simulink model "dmt_sim"  (Simulink 6.0)
settings: Solver=ode45  StartTime=0.0  StopTime=inf  RelTol=1e-3
model workspace: external: M-Code (data not in the file)
undefined symbols (not defined in the file or in its folder): b, slcm
libraries: commdigbbndam2 x512, simulink x35, dspxfrm3 x2, commchan2 x1, commrandsrc2 x1, dspsigattribs x1, dspsrcs4 x1, dspindex x1, commsink2 x1, dspsnks4 x1
(part 5 of 5)

== system dmt_sim/DMT Modulator/Modulator Bank 6 ==
  In1 : Inport  LatchInput=off
  Demux1 : Demux  Outputs=b(offset+1:offset+16)
  Matrix Concatenation : simulink/Math Operations/Matrix Concatenation  numInports=16  catMethod=Vertical
  Rectangular QAM Modulator Baseband1 : commdigbbndam2/Rectangular QAM Modulator Baseband  M=2^b(offset+1)  InType=Bit  Enc=Binary  PowType=Min. distance between symbols  MinDist=2  AvgPow=1  PeakPow=1  Ph=0  numSamp=1
  Rectangular QAM Modulator Baseband10 : commdigbbndam2/Rectangular QAM Modulator Baseband  M=2^b(offset+10)  InType=Bit  Enc=Binary  PowType=Min. distance between symbols  MinDist=2  AvgPow=1  PeakPow=1  Ph=0  numSamp=1
  Rectangular QAM Modulator Baseband11 : commdigbbndam2/Rectangular QAM Modulator Baseband  M=2^b(offset+11)  InType=Bit  Enc=Binary  PowType=Min. distance between symbols  MinDist=2  AvgPow=1  PeakPow=1  Ph=0  numSamp=1
  Rectangular QAM Modulator Baseband12 : commdigbbndam2/Rectangular QAM Modulator Baseband  M=2^b(offset+12)  InType=Bit  Enc=Binary  PowType=Min. distance between symbols  MinDist=2  AvgPow=1  PeakPow=1  Ph=0  numSamp=1
  Rectangular QAM Modulator Baseband13 : commdigbbndam2/Rectangular QAM Modulator Baseband  M=2^b(offset+13)  InType=Bit  Enc=Binary  PowType=Min. distance between symbols  MinDist=2  AvgPow=1  PeakPow=1  Ph=0  numSamp=1
  Rectangular QAM Modulator Baseband14 : commdigbbndam2/Rectangular QAM Modulator Baseband  M=2^b(offset+14)  InType=Bit  Enc=Binary  PowType=Min. distance between symbols  MinDist=2  AvgPow=1  PeakPow=1  Ph=0  numSamp=1
  Rectangular QAM Modulator Baseband15 : commdigbbndam2/Rectangular QAM Modulator Baseband  M=2^b(offset+15)  InType=Bit  Enc=Binary  PowType=Min. distance between symbols  MinDist=2  AvgPow=1  PeakPow=1  Ph=0  numSamp=1
  Rectangular QAM Modulator Baseband16 : commdigbbndam2/Rectangular QAM Modulator Baseband  M=2^b(offset+16)  InType=Bit  Enc=Binary  PowType=Min. distance between symbols  MinDist=2  AvgPow=1  PeakPow=1  Ph=0  numSamp=1
  Rectangular QAM Modulator Baseband2 : commdigbbndam2/Rectangular QAM Modulator Baseband  M=2^b(offset+2)  InType=Bit  Enc=Binary  PowType=Min. distance between symbols  MinDist=2  AvgPow=1  PeakPow=1  Ph=0  numSamp=1
  Rectangular QAM Modulator Baseband3 : commdigbbndam2/Rectangular QAM Modulator Baseband  M=2^b(offset+3)  InType=Bit  Enc=Binary  PowType=Min. distance between symbols  MinDist=2  AvgPow=1  PeakPow=1  Ph=0  numSamp=1
  Rectangular QAM Modulator Baseband4 : commdigbbndam2/Rectangular QAM Modulator Baseband  M=2^b(offset+4)  InType=Bit  Enc=Binary  PowType=Min. distance between symbols  MinDist=2  AvgPow=1  PeakPow=1  Ph=0  numSamp=1
  Rectangular QAM Modulator Baseband5 : commdigbbndam2/Rectangular QAM Modulator Baseband  M=2^b(offset+5)  InType=Bit  Enc=Binary  PowType=Min. distance between symbols  MinDist=2  AvgPow=1  PeakPow=1  Ph=0  numSamp=1
  Rectangular QAM Modulator Baseband6 : commdigbbndam2/Rectangular QAM Modulator Baseband  M=2^b(offset+6)  InType=Bit  Enc=Binary  PowType=Min. distance between symbols  MinDist=2  AvgPow=1  PeakPow=1  Ph=0  numSamp=1
  Rectangular QAM Modulator Baseband7 : commdigbbndam2/Rectangular QAM Modulator Baseband  M=2^b(offset+7)  InType=Bit  Enc=Binary  PowType=Min. distance between symbols  MinDist=2  AvgPow=1  PeakPow=1  Ph=0  numSamp=1
  Rectangular QAM Modulator Baseband8 : commdigbbndam2/Rectangular QAM Modulator Baseband  M=2^b(offset+8)  InType=Bit  Enc=Binary  PowType=Min. distance between symbols  MinDist=2  AvgPow=1  PeakPow=1  Ph=0  numSamp=1
  Rectangular QAM Modulator Baseband9 : commdigbbndam2/Rectangular QAM Modulator Baseband  M=2^b(offset+9)  InType=Bit  Enc=Binary  PowType=Min. distance between symbols  MinDist=2  AvgPow=1  PeakPow=1  Ph=0  numSamp=1
  Out1 : Outport
  wires:
  Rectangular QAM Modulator Baseband16/1 -> Matrix Concatenation/16
  Rectangular QAM Modulator Baseband15/1 -> Matrix Concatenation/15
  Rectangular QAM Modulator Baseband14/1 -> Matrix Concatenation/14
  Rectangular QAM Modulator Baseband13/1 -> Matrix Concatenation/13
  Rectangular QAM Modulator Baseband12/1 -> Matrix Concatenation/12
  Rectangular QAM Modulator Baseband11/1 -> Matrix Concatenation/11
  Rectangular QAM Modulator Baseband10/1 -> Matrix Concatenation/10
  Rectangular QAM Modulator Baseband9/1 -> Matrix Concatenation/9
  Rectangular QAM Modulator Baseband8/1 -> Matrix Concatenation/8
  Rectangular QAM Modulator Baseband7/1 -> Matrix Concatenation/7
  Rectangular QAM Modulator Baseband6/1 -> Matrix Concatenation/6
  Rectangular QAM Modulator Baseband5/1 -> Matrix Concatenation/5
  Rectangular QAM Modulator Baseband4/1 -> Matrix Concatenation/4
  Rectangular QAM Modulator Baseband3/1 -> Matrix Concatenation/3
  Rectangular QAM Modulator Baseband2/1 -> Matrix Concatenation/2
  Demux1/16 -> Rectangular QAM Modulator Baseband16/1
  Demux1/15 -> Rectangular QAM Modulator Baseband15/1
  Demux1/14 -> Rectangular QAM Modulator Baseband14/1
  Demux1/13 -> Rectangular QAM Modulator Baseband13/1
  Demux1/12 -> Rectangular QAM Modulator Baseband12/1
  Demux1/11 -> Rectangular QAM Modulator Baseband11/1
  Demux1/10 -> Rectangular QAM Modulator Baseband10/1
  Demux1/9 -> Rectangular QAM Modulator Baseband9/1
  Demux1/8 -> Rectangular QAM Modulator Baseband8/1
  Demux1/7 -> Rectangular QAM Modulator Baseband7/1
  Demux1/6 -> Rectangular QAM Modulator Baseband6/1
  Demux1/5 -> Rectangular QAM Modulator Baseband5/1
  Demux1/4 -> Rectangular QAM Modulator Baseband4/1
  Demux1/3 -> Rectangular QAM Modulator Baseband3/1
  Matrix Concatenation/1 -> Out1/1
  In1/1 -> Demux1/1
  Demux1/2 -> Rectangular QAM Modulator Baseband2/1
  Demux1/1 -> Rectangular QAM Modulator Baseband1/1
  Rectangular QAM Modulator Baseband1/1 -> Matrix Concatenation/1

== system dmt_sim/DMT Modulator/Modulator Bank 7 ==
  In1 : Inport  LatchInput=off
  Demux1 : Demux  Outputs=b(offset+1:offset+16)
  Matrix Concatenation : simulink/Math Operations/Matrix Concatenation  numInports=16  catMethod=Vertical
  Rectangular QAM Modulator Baseband1 : commdigbbndam2/Rectangular QAM Modulator Baseband  M=2^b(offset+1)  InType=Bit  Enc=Binary  PowType=Min. distance between symbols  MinDist=2  AvgPow=1  PeakPow=1  Ph=0  numSamp=1
  Rectangular QAM Modulator Baseband10 : commdigbbndam2/Rectangular QAM Modulator Baseband  M=2^b(offset+10)  InType=Bit  Enc=Binary  PowType=Min. distance between symbols  MinDist=2  AvgPow=1  PeakPow=1  Ph=0  numSamp=1
  Rectangular QAM Modulator Baseband11 : commdigbbndam2/Rectangular QAM Modulator Baseband  M=2^b(offset+11)  InType=Bit  Enc=Binary  PowType=Min. distance between symbols  MinDist=2  AvgPow=1  PeakPow=1  Ph=0  numSamp=1
  Rectangular QAM Modulator Baseband12 : commdigbbndam2/Rectangular QAM Modulator Baseband  M=2^b(offset+12)  InType=Bit  Enc=Binary  PowType=Min. distance between symbols  MinDist=2  AvgPow=1  PeakPow=1  Ph=0  numSamp=1
  Rectangular QAM Modulator Baseband13 : commdigbbndam2/Rectangular QAM Modulator Baseband  M=2^b(offset+13)  InType=Bit  Enc=Binary  PowType=Min. distance between symbols  MinDist=2  AvgPow=1  PeakPow=1  Ph=0  numSamp=1
  Rectangular QAM Modulator Baseband14 : commdigbbndam2/Rectangular QAM Modulator Baseband  M=2^b(offset+14)  InType=Bit  Enc=Binary  PowType=Min. distance between symbols  MinDist=2  AvgPow=1  PeakPow=1  Ph=0  numSamp=1
  Rectangular QAM Modulator Baseband15 : commdigbbndam2/Rectangular QAM Modulator Baseband  M=2^b(offset+15)  InType=Bit  Enc=Binary  PowType=Min. distance between symbols  MinDist=2  AvgPow=1  PeakPow=1  Ph=0  numSamp=1
  Rectangular QAM Modulator Baseband16 : commdigbbndam2/Rectangular QAM Modulator Baseband  M=2^b(offset+16)  InType=Bit  Enc=Binary  PowType=Min. distance between symbols  MinDist=2  AvgPow=1  PeakPow=1  Ph=0  numSamp=1
  Rectangular QAM Modulator Baseband2 : commdigbbndam2/Rectangular QAM Modulator Baseband  M=2^b(offset+2)  InType=Bit  Enc=Binary  PowType=Min. distance between symbols  MinDist=2  AvgPow=1  PeakPow=1  Ph=0  numSamp=1
  Rectangular QAM Modulator Baseband3 : commdigbbndam2/Rectangular QAM Modulator Baseband  M=2^b(offset+3)  InType=Bit  Enc=Binary  PowType=Min. distance between symbols  MinDist=2  AvgPow=1  PeakPow=1  Ph=0  numSamp=1
  Rectangular QAM Modulator Baseband4 : commdigbbndam2/Rectangular QAM Modulator Baseband  M=2^b(offset+4)  InType=Bit  Enc=Binary  PowType=Min. distance between symbols  MinDist=2  AvgPow=1  PeakPow=1  Ph=0  numSamp=1
  Rectangular QAM Modulator Baseband5 : commdigbbndam2/Rectangular QAM Modulator Baseband  M=2^b(offset+5)  InType=Bit  Enc=Binary  PowType=Min. distance between symbols  MinDist=2  AvgPow=1  PeakPow=1  Ph=0  numSamp=1
  Rectangular QAM Modulator Baseband6 : commdigbbndam2/Rectangular QAM Modulator Baseband  M=2^b(offset+6)  InType=Bit  Enc=Binary  PowType=Min. distance between symbols  MinDist=2  AvgPow=1  PeakPow=1  Ph=0  numSamp=1
  Rectangular QAM Modulator Baseband7 : commdigbbndam2/Rectangular QAM Modulator Baseband  M=2^b(offset+7)  InType=Bit  Enc=Binary  PowType=Min. distance between symbols  MinDist=2  AvgPow=1  PeakPow=1  Ph=0  numSamp=1
  Rectangular QAM Modulator Baseband8 : commdigbbndam2/Rectangular QAM Modulator Baseband  M=2^b(offset+8)  InType=Bit  Enc=Binary  PowType=Min. distance between symbols  MinDist=2  AvgPow=1  PeakPow=1  Ph=0  numSamp=1
  Rectangular QAM Modulator Baseband9 : commdigbbndam2/Rectangular QAM Modulator Baseband  M=2^b(offset+9)  InType=Bit  Enc=Binary  PowType=Min. distance between symbols  MinDist=2  AvgPow=1  PeakPow=1  Ph=0  numSamp=1
  Out1 : Outport
  wires:
  Rectangular QAM Modulator Baseband1/1 -> Matrix Concatenation/1
  Demux1/1 -> Rectangular QAM Modulator Baseband1/1
  Demux1/2 -> Rectangular QAM Modulator Baseband2/1
  In1/1 -> Demux1/1
  Matrix Concatenation/1 -> Out1/1
  Demux1/3 -> Rectangular QAM Modulator Baseband3/1
  Demux1/4 -> Rectangular QAM Modulator Baseband4/1
  Demux1/5 -> Rectangular QAM Modulator Baseband5/1
  Demux1/6 -> Rectangular QAM Modulator Baseband6/1
  Demux1/7 -> Rectangular QAM Modulator Baseband7/1
  Demux1/8 -> Rectangular QAM Modulator Baseband8/1
  Demux1/9 -> Rectangular QAM Modulator Baseband9/1
  Demux1/10 -> Rectangular QAM Modulator Baseband10/1
  Demux1/11 -> Rectangular QAM Modulator Baseband11/1
  Demux1/12 -> Rectangular QAM Modulator Baseband12/1
  Demux1/13 -> Rectangular QAM Modulator Baseband13/1
  Demux1/14 -> Rectangular QAM Modulator Baseband14/1
  Demux1/15 -> Rectangular QAM Modulator Baseband15/1
  Demux1/16 -> Rectangular QAM Modulator Baseband16/1
  Rectangular QAM Modulator Baseband2/1 -> Matrix Concatenation/2
  Rectangular QAM Modulator Baseband3/1 -> Matrix Concatenation/3
  Rectangular QAM Modulator Baseband4/1 -> Matrix Concatenation/4
  Rectangular QAM Modulator Baseband5/1 -> Matrix Concatenation/5
  Rectangular QAM Modulator Baseband6/1 -> Matrix Concatenation/6
  Rectangular QAM Modulator Baseband7/1 -> Matrix Concatenation/7
  Rectangular QAM Modulator Baseband8/1 -> Matrix Concatenation/8
  Rectangular QAM Modulator Baseband9/1 -> Matrix Concatenation/9
  Rectangular QAM Modulator Baseband10/1 -> Matrix Concatenation/10
  Rectangular QAM Modulator Baseband11/1 -> Matrix Concatenation/11
  Rectangular QAM Modulator Baseband12/1 -> Matrix Concatenation/12
  Rectangular QAM Modulator Baseband13/1 -> Matrix Concatenation/13
  Rectangular QAM Modulator Baseband14/1 -> Matrix Concatenation/14
  Rectangular QAM Modulator Baseband15/1 -> Matrix Concatenation/15
  Rectangular QAM Modulator Baseband16/1 -> Matrix Concatenation/16

== system dmt_sim/DMT Modulator/Modulator Bank 8 ==
  In1 : Inport  LatchInput=off
  Demux1 : Demux  Outputs=b(offset+1:offset+16)
  Matrix Concatenation : simulink/Math Operations/Matrix Concatenation  numInports=16  catMethod=Vertical
  Rectangular QAM Modulator Baseband1 : commdigbbndam2/Rectangular QAM Modulator Baseband  M=2^b(offset+1)  InType=Bit  Enc=Binary  PowType=Min. distance between symbols  MinDist=2  AvgPow=1  PeakPow=1  Ph=0  numSamp=1
  Rectangular QAM Modulator Baseband10 : commdigbbndam2/Rectangular QAM Modulator Baseband  M=2^b(offset+10)  InType=Bit  Enc=Binary  PowType=Min. distance between symbols  MinDist=2  AvgPow=1  PeakPow=1  Ph=0  numSamp=1
  Rectangular QAM Modulator Baseband11 : commdigbbndam2/Rectangular QAM Modulator Baseband  M=2^b(offset+11)  InType=Bit  Enc=Binary  PowType=Min. distance between symbols  MinDist=2  AvgPow=1  PeakPow=1  Ph=0  numSamp=1
  Rectangular QAM Modulator Baseband12 : commdigbbndam2/Rectangular QAM Modulator Baseband  M=2^b(offset+12)  InType=Bit  Enc=Binary  PowType=Min. distance between symbols  MinDist=2  AvgPow=1  PeakPow=1  Ph=0  numSamp=1
  Rectangular QAM Modulator Baseband13 : commdigbbndam2/Rectangular QAM Modulator Baseband  M=2^b(offset+13)  InType=Bit  Enc=Binary  PowType=Min. distance between symbols  MinDist=2  AvgPow=1  PeakPow=1  Ph=0  numSamp=1
  Rectangular QAM Modulator Baseband14 : commdigbbndam2/Rectangular QAM Modulator Baseband  M=2^b(offset+14)  InType=Bit  Enc=Binary  PowType=Min. distance between symbols  MinDist=2  AvgPow=1  PeakPow=1  Ph=0  numSamp=1
  Rectangular QAM Modulator Baseband15 : commdigbbndam2/Rectangular QAM Modulator Baseband  M=2^b(offset+15)  InType=Bit  Enc=Binary  PowType=Min. distance between symbols  MinDist=2  AvgPow=1  PeakPow=1  Ph=0  numSamp=1
  Rectangular QAM Modulator Baseband16 : commdigbbndam2/Rectangular QAM Modulator Baseband  M=2^b(offset+16)  InType=Bit  Enc=Binary  PowType=Min. distance between symbols  MinDist=2  AvgPow=1  PeakPow=1  Ph=0  numSamp=1
  Rectangular QAM Modulator Baseband2 : commdigbbndam2/Rectangular QAM Modulator Baseband  M=2^b(offset+2)  InType=Bit  Enc=Binary  PowType=Min. distance between symbols  MinDist=2  AvgPow=1  PeakPow=1  Ph=0  numSamp=1
  Rectangular QAM Modulator Baseband3 : commdigbbndam2/Rectangular QAM Modulator Baseband  M=2^b(offset+3)  InType=Bit  Enc=Binary  PowType=Min. distance between symbols  MinDist=2  AvgPow=1  PeakPow=1  Ph=0  numSamp=1
  Rectangular QAM Modulator Baseband4 : commdigbbndam2/Rectangular QAM Modulator Baseband  M=2^b(offset+4)  InType=Bit  Enc=Binary  PowType=Min. distance between symbols  MinDist=2  AvgPow=1  PeakPow=1  Ph=0  numSamp=1
  Rectangular QAM Modulator Baseband5 : commdigbbndam2/Rectangular QAM Modulator Baseband  M=2^b(offset+5)  InType=Bit  Enc=Binary  PowType=Min. distance between symbols  MinDist=2  AvgPow=1  PeakPow=1  Ph=0  numSamp=1
  Rectangular QAM Modulator Baseband6 : commdigbbndam2/Rectangular QAM Modulator Baseband  M=2^b(offset+6)  InType=Bit  Enc=Binary  PowType=Min. distance between symbols  MinDist=2  AvgPow=1  PeakPow=1  Ph=0  numSamp=1
  Rectangular QAM Modulator Baseband7 : commdigbbndam2/Rectangular QAM Modulator Baseband  M=2^b(offset+7)  InType=Bit  Enc=Binary  PowType=Min. distance between symbols  MinDist=2  AvgPow=1  PeakPow=1  Ph=0  numSamp=1
  Rectangular QAM Modulator Baseband8 : commdigbbndam2/Rectangular QAM Modulator Baseband  M=2^b(offset+8)  InType=Bit  Enc=Binary  PowType=Min. distance between symbols  MinDist=2  AvgPow=1  PeakPow=1  Ph=0  numSamp=1
  Rectangular QAM Modulator Baseband9 : commdigbbndam2/Rectangular QAM Modulator Baseband  M=2^b(offset+9)  InType=Bit  Enc=Binary  PowType=Min. distance between symbols  MinDist=2  AvgPow=1  PeakPow=1  Ph=0  numSamp=1
  Out1 : Outport
  wires:
  Rectangular QAM Modulator Baseband16/1 -> Matrix Concatenation/16
  Rectangular QAM Modulator Baseband15/1 -> Matrix Concatenation/15
  Rectangular QAM Modulator Baseband14/1 -> Matrix Concatenation/14
  Rectangular QAM Modulator Baseband13/1 -> Matrix Concatenation/13
  Rectangular QAM Modulator Baseband12/1 -> Matrix Concatenation/12
  Rectangular QAM Modulator Baseband11/1 -> Matrix Concatenation/11
  Rectangular QAM Modulator Baseband10/1 -> Matrix Concatenation/10
  Rectangular QAM Modulator Baseband9/1 -> Matrix Concatenation/9
  Rectangular QAM Modulator Baseband8/1 -> Matrix Concatenation/8
  Rectangular QAM Modulator Baseband7/1 -> Matrix Concatenation/7
  Rectangular QAM Modulator Baseband6/1 -> Matrix Concatenation/6
  Rectangular QAM Modulator Baseband5/1 -> Matrix Concatenation/5
  Rectangular QAM Modulator Baseband4/1 -> Matrix Concatenation/4
  Rectangular QAM Modulator Baseband3/1 -> Matrix Concatenation/3
  Rectangular QAM Modulator Baseband2/1 -> Matrix Concatenation/2
  Demux1/16 -> Rectangular QAM Modulator Baseband16/1
  Demux1/15 -> Rectangular QAM Modulator Baseband15/1
  Demux1/14 -> Rectangular QAM Modulator Baseband14/1
  Demux1/13 -> Rectangular QAM Modulator Baseband13/1
  Demux1/12 -> Rectangular QAM Modulator Baseband12/1
  Demux1/11 -> Rectangular QAM Modulator Baseband11/1
  Demux1/10 -> Rectangular QAM Modulator Baseband10/1
  Demux1/9 -> Rectangular QAM Modulator Baseband9/1
  Demux1/8 -> Rectangular QAM Modulator Baseband8/1
  Demux1/7 -> Rectangular QAM Modulator Baseband7/1
  Demux1/6 -> Rectangular QAM Modulator Baseband6/1
  Demux1/5 -> Rectangular QAM Modulator Baseband5/1
  Demux1/4 -> Rectangular QAM Modulator Baseband4/1
  Demux1/3 -> Rectangular QAM Modulator Baseband3/1
  Matrix Concatenation/1 -> Out1/1
  In1/1 -> Demux1/1
  Demux1/2 -> Rectangular QAM Modulator Baseband2/1
  Demux1/1 -> Rectangular QAM Modulator Baseband1/1
  Rectangular QAM Modulator Baseband1/1 -> Matrix Concatenation/1

== system dmt_sim/DMT Modulator/Modulator Bank 9 ==
  In1 : Inport  LatchInput=off
  Demux1 : Demux  Outputs=b(offset+1:offset+16)
  Matrix Concatenation : simulink/Math Operations/Matrix Concatenation  numInports=16  catMethod=Vertical
  Rectangular QAM Modulator Baseband1 : commdigbbndam2/Rectangular QAM Modulator Baseband  M=2^b(offset+1)  InType=Bit  Enc=Binary  PowType=Min. distance between symbols  MinDist=2  AvgPow=1  PeakPow=1  Ph=0  numSamp=1
  Rectangular QAM Modulator Baseband10 : commdigbbndam2/Rectangular QAM Modulator Baseband  M=2^b(offset+10)  InType=Bit  Enc=Binary  PowType=Min. distance between symbols  MinDist=2  AvgPow=1  PeakPow=1  Ph=0  numSamp=1
  Rectangular QAM Modulator Baseband11 : commdigbbndam2/Rectangular QAM Modulator Baseband  M=2^b(offset+11)  InType=Bit  Enc=Binary  PowType=Min. distance between symbols  MinDist=2  AvgPow=1  PeakPow=1  Ph=0  numSamp=1
  Rectangular QAM Modulator Baseband12 : commdigbbndam2/Rectangular QAM Modulator Baseband  M=2^b(offset+12)  InType=Bit  Enc=Binary  PowType=Min. distance between symbols  MinDist=2  AvgPow=1  PeakPow=1  Ph=0  numSamp=1
  Rectangular QAM Modulator Baseband13 : commdigbbndam2/Rectangular QAM Modulator Baseband  M=2^b(offset+13)  InType=Bit  Enc=Binary  PowType=Min. distance between symbols  MinDist=2  AvgPow=1  PeakPow=1  Ph=0  numSamp=1
  Rectangular QAM Modulator Baseband14 : commdigbbndam2/Rectangular QAM Modulator Baseband  M=2^b(offset+14)  InType=Bit  Enc=Binary  PowType=Min. distance between symbols  MinDist=2  AvgPow=1  PeakPow=1  Ph=0  numSamp=1
  Rectangular QAM Modulator Baseband15 : commdigbbndam2/Rectangular QAM Modulator Baseband  M=2^b(offset+15)  InType=Bit  Enc=Binary  PowType=Min. distance between symbols  MinDist=2  AvgPow=1  PeakPow=1  Ph=0  numSamp=1
  Rectangular QAM Modulator Baseband16 : commdigbbndam2/Rectangular QAM Modulator Baseband  M=2^b(offset+16)  InType=Bit  Enc=Binary  PowType=Min. distance between symbols  MinDist=2  AvgPow=1  PeakPow=1  Ph=0  numSamp=1
  Rectangular QAM Modulator Baseband2 : commdigbbndam2/Rectangular QAM Modulator Baseband  M=2^b(offset+2)  InType=Bit  Enc=Binary  PowType=Min. distance between symbols  MinDist=2  AvgPow=1  PeakPow=1  Ph=0  numSamp=1
  Rectangular QAM Modulator Baseband3 : commdigbbndam2/Rectangular QAM Modulator Baseband  M=2^b(offset+3)  InType=Bit  Enc=Binary  PowType=Min. distance between symbols  MinDist=2  AvgPow=1  PeakPow=1  Ph=0  numSamp=1
  Rectangular QAM Modulator Baseband4 : commdigbbndam2/Rectangular QAM Modulator Baseband  M=2^b(offset+4)  InType=Bit  Enc=Binary  PowType=Min. distance between symbols  MinDist=2  AvgPow=1  PeakPow=1  Ph=0  numSamp=1
  Rectangular QAM Modulator Baseband5 : commdigbbndam2/Rectangular QAM Modulator Baseband  M=2^b(offset+5)  InType=Bit  Enc=Binary  PowType=Min. distance between symbols  MinDist=2  AvgPow=1  PeakPow=1  Ph=0  numSamp=1
  Rectangular QAM Modulator Baseband6 : commdigbbndam2/Rectangular QAM Modulator Baseband  M=2^b(offset+6)  InType=Bit  Enc=Binary  PowType=Min. distance between symbols  MinDist=2  AvgPow=1  PeakPow=1  Ph=0  numSamp=1
  Rectangular QAM Modulator Baseband7 : commdigbbndam2/Rectangular QAM Modulator Baseband  M=2^b(offset+7)  InType=Bit  Enc=Binary  PowType=Min. distance between symbols  MinDist=2  AvgPow=1  PeakPow=1  Ph=0  numSamp=1
  Rectangular QAM Modulator Baseband8 : commdigbbndam2/Rectangular QAM Modulator Baseband  M=2^b(offset+8)  InType=Bit  Enc=Binary  PowType=Min. distance between symbols  MinDist=2  AvgPow=1  PeakPow=1  Ph=0  numSamp=1
  Rectangular QAM Modulator Baseband9 : commdigbbndam2/Rectangular QAM Modulator Baseband  M=2^b(offset+9)  InType=Bit  Enc=Binary  PowType=Min. distance between symbols  MinDist=2  AvgPow=1  PeakPow=1  Ph=0  numSamp=1
  Out1 : Outport
  wires:
  Rectangular QAM Modulator Baseband1/1 -> Matrix Concatenation/1
  Demux1/1 -> Rectangular QAM Modulator Baseband1/1
  Demux1/2 -> Rectangular QAM Modulator Baseband2/1
  In1/1 -> Demux1/1
  Matrix Concatenation/1 -> Out1/1
  Demux1/3 -> Rectangular QAM Modulator Baseband3/1
  Demux1/4 -> Rectangular QAM Modulator Baseband4/1
  Demux1/5 -> Rectangular QAM Modulator Baseband5/1
  Demux1/6 -> Rectangular QAM Modulator Baseband6/1
  Demux1/7 -> Rectangular QAM Modulator Baseband7/1
  Demux1/8 -> Rectangular QAM Modulator Baseband8/1
  Demux1/9 -> Rectangular QAM Modulator Baseband9/1
  Demux1/10 -> Rectangular QAM Modulator Baseband10/1
  Demux1/11 -> Rectangular QAM Modulator Baseband11/1
  Demux1/12 -> Rectangular QAM Modulator Baseband12/1
  Demux1/13 -> Rectangular QAM Modulator Baseband13/1
  Demux1/14 -> Rectangular QAM Modulator Baseband14/1
  Demux1/15 -> Rectangular QAM Modulator Baseband15/1
  Demux1/16 -> Rectangular QAM Modulator Baseband16/1
  Rectangular QAM Modulator Baseband2/1 -> Matrix Concatenation/2
  Rectangular QAM Modulator Baseband3/1 -> Matrix Concatenation/3
  Rectangular QAM Modulator Baseband4/1 -> Matrix Concatenation/4
  Rectangular QAM Modulator Baseband5/1 -> Matrix Concatenation/5
  Rectangular QAM Modulator Baseband6/1 -> Matrix Concatenation/6
  Rectangular QAM Modulator Baseband7/1 -> Matrix Concatenation/7
  Rectangular QAM Modulator Baseband8/1 -> Matrix Concatenation/8
  Rectangular QAM Modulator Baseband9/1 -> Matrix Concatenation/9
  Rectangular QAM Modulator Baseband10/1 -> Matrix Concatenation/10
  Rectangular QAM Modulator Baseband11/1 -> Matrix Concatenation/11
  Rectangular QAM Modulator Baseband12/1 -> Matrix Concatenation/12
  Rectangular QAM Modulator Baseband13/1 -> Matrix Concatenation/13
  Rectangular QAM Modulator Baseband14/1 -> Matrix Concatenation/14
  Rectangular QAM Modulator Baseband15/1 -> Matrix Concatenation/15
  Rectangular QAM Modulator Baseband16/1 -> Matrix Concatenation/16

== system dmt_sim/Model Info/EmptySubsystem ==
